simulink model "G_actuatordynamics"  (R2017a)
settings: Solver=FixedStepAuto  StartTime=0.0  StopTime=10  FixedStep=sim_time  RelTol=1e-3  EnableMultiTasking=on
values from neighbouring files (symbols this model uses):
  B = [1 0.5 -0.5 -1 0 0.5 ; 0 0 0 0 2 0 ; -0.05 -0.02 0.02 0.05 0 2 ; -1 -1 -1 -1 -2 0]    [A_runSimulation.m]    (also in C_runSimulation.m; D_runSimulation.m; E_runSimulation.m; F_runSimulation.m)
  gain_four = rand()*2    [A_runSimulation.m]    (also in C_runSimulation.m = 0; D_runSimulation.m; E_runSimulation.m = 0; F_runSimulation.m = 0)
  gain_one = rand()*2    [A_runSimulation.m]    (also in C_runSimulation.m = 0; D_runSimulation.m; E_runSimulation.m = 0; F_runSimulation.m = 0)
  gain_three = rand()*2    [A_runSimulation.m]    (also in C_runSimulation.m = 0; D_runSimulation.m; E_runSimulation.m = 0; F_runSimulation.m = 0)
  gain_two = rand()*2    [A_runSimulation.m]    (also in C_runSimulation.m = 0; D_runSimulation.m; E_runSimulation.m = 0; F_runSimulation.m = 0)
  seed_four = k + 30    [A_runSimulation.m]    (also in C_runSimulation.m; D_runSimulation.m; E_runSimulation.m; F_runSimulation.m)
  seed_one = k    [A_runSimulation.m]    (also in C_runSimulation.m; D_runSimulation.m; E_runSimulation.m; F_runSimulation.m)
  seed_three = k + 20    [A_runSimulation.m]    (also in C_runSimulation.m; D_runSimulation.m; E_runSimulation.m; F_runSimulation.m)
  seed_two = k + 10    [A_runSimulation.m]    (also in C_runSimulation.m; D_runSimulation.m; E_runSimulation.m; F_runSimulation.m)
  signal_gain = j    [A_runSimulation.m]    (also in C_runSimulation.m; D_runSimulation.m; E_runSimulation.m = 0.3; F_runSimulation.m)
  sim_time = 1    [E_runSimulation.m]    (also in F_runSimulation.m = 0.1; F_runSimulation2.m = 0.1; G_runSimulation.m = 0.001)
  u_lim = [[-0.5 -0.5 -0.5 -0.5 -0.5 -0.5]' [0.5 0.5 0.5 0.5 0.5 0.5]']    [A_runSimulation.m]    (also in C_runSimulation.m; D_runSimulation.m; E_runSimulation.m; F_runSimulation.m)
  udot_lim = [[2 2 2 2 2 2]']    [A_runSimulation.m]    (also in C_runSimulation.m; D_runSimulation.m; E_runSimulation.m; F_runSimulation.m)
  W1 = eye(6)    [G_runSimulation.m]
  W2 = eye(6)    [G_runSimulation.m]
libraries: dspsrcs4 x8
(part 2 of 2)

== matlab function G_actuatordynamics/FRAMEWISE CONTROL ALLOCATION simple pseudoinverse4/Pseudoinverse1 ==
  data: mdes input; xdot_prev input; u output; B input; A input; dt input; W1 input; W2 input; u_lim input; reductionType input; saturated output
function [u, saturated] = Pseudoinverse(mdes, xdot_prev, B, A, dt, W1, W2, u_lim, reductionType)
coder.varsize('u_index', 'Br', 'Wr', 'u_sat');

%check if the matrices are correct
    if not(isequal(size(u_lim,1),size(B,2),size(W1,1),size(W1,2),size(W2,1),size(W2,2))...
       && isequal(size(mdes,1),size(B,1),size(A,1),size(A,2),size(xdot_prev,1)))
        error ('input matrix dimensions do not match')
    end
    
%assign to every equation an index    
    u_index = [1:length(u_lim)].';
    I = eye(length(xdot_prev));
    
%compute the remaining moment to compensate
    m = mdes - (I + A*dt)*xdot_prev;
    
%check the type of system and then compute the pseudoinverse 1st step
    order = size(B,2)-size(B,1);

    if order > 0 %over-determined, solution that minimizes the 2norm
        W = power((power(W1,2) + power(W2,2)),1/2);
        H = B*inv(W);
        G = inv(W) * (H'*inv(H*H'));
        II = eye(size(G*B,1));
        F = (II - G*B)*power(inv(W),2)*power(W2,2);
        u = inv(W)*B'*inv(B*inv(W)*B')*m;
    elseif order < 0 %under-determined, solution that minimizes the error
        u = inv(B'*B)*B'*m;   
    else %order = 0, sqared thus invertiBrle
        u = inv(B)*m;
    end

%deifne u_sat vector
    u_sat = zeros(length(u),1);
    
    saturated = 0;
%check if the first iteration solution is correct then return    
    if not(any(u <= u_lim(:,1))||any(u >= u_lim(:,2)))  
        return
    end
    
    saturated = 1;
%The software continues only if the solution has to be reduced
%reduce their value
    switch reductionType
        case 1 %truncation
            %takes note of which one are out of their bounds
                u_sat(u < u_lim(:,1)) = 1;
                u_sat(u > u_lim(:,2)) = 1;
                
            %trucate
                u = min(u, u_lim(:,2));
                u = max(u, u_lim(:,1));

        case 2 %scaling solution -> direction preserving
            %reduce
                a = zeros(length(u),1);

                for i = 1:length(u)
                    if u(i)>0
                       a(i) = abs(u(i)/u_lim(i,2));
                    elseif u(i)<0
                       a(i) = abs(u(i)/u_lim(i,1));
                    else
                       a(i) = 0; 
                    end          
                end
                a_max = max(a);
                a_max = max(a_max,1);
                u = u/a_max;
            
            %takes note of which one are out of their bounds
                u_sat(u == u_lim(:,2)) = 1;
                u_sat(u == u_lim(:,1)) = 1;
            
    end
    
return
    
end

== matlab function G_actuatordynamics/error6 ==
  data: e input; error output
function error = error(e)

    error = sum(abs(e));

end
